simulink model "TOAD_Controller"  (R2025b)
settings: Solver=VariableStepAuto  StartTime=0.0  StopTime=10.0  RelTol=1e-3
undefined symbols (not defined in the file or in its folder): constantsASTRA, dt_SIM, u0
settings Model: Creator=pplat  LastModifiedBy=andrew

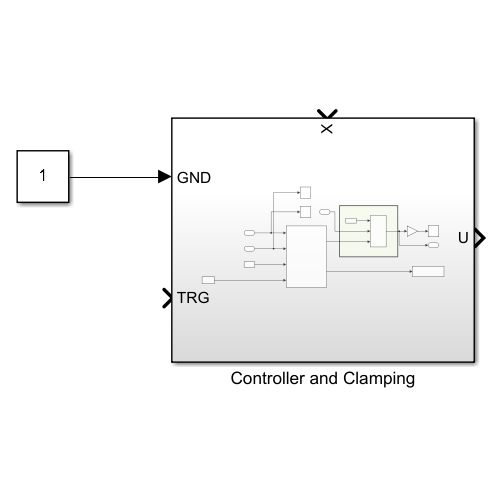
[thumbnail: Simulink's stored preview of the top-level diagram]
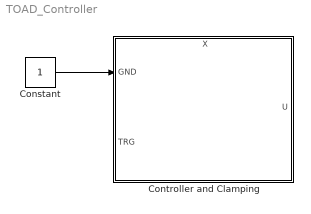
== system TOAD_Controller ==
  Constant : Constant
  Controller and Clamping : Subsystem
      settings: PortSchema="{\"entries\":[{\"content\":{\"sides\":[{\"content\":{\"connectorIds\":[\"In1\",\"In2\"]},\"type\":\"ConnectorPlacement.EquallySpacedRectSide\",\"uuid\":\"ecbe546b-cb94-472f-8bff-97599afc2d8a\"},{\"content\":{\"connectorIds\":[\"Out1\"],\"side\":\"RIGHT\"},\"type\":\"ConnectorPlacement.EquallySpacedRectSide\",\"uuid\":\"5863f614-a2a8-49af-9209-63f06ca85da1\"},{\"content\":{\"connectorIds\":[\"In3\"],\"side\":\"TOP\"},\"type\":\"ConnectorPlacement.EquallySpacedRectSide\",\"uuid\":\"6e100a99-a304-4bec-8fe0-0dacf7d0f0e2\"}]},\"type\":\"ConnectorPlacement.EquallySpacedConnector\",\"uuid\":\"0527d0f7-8d45-4b0a-99f9-95f3ca68c54e\"}],\"packageUris\":[\"http://schema.mathworks.com/mf0/Connector/R2020b\"],\"version\":\"1.0\"}"
  wires:
  Constant/1 -> Controller and Clamping/1(GND)

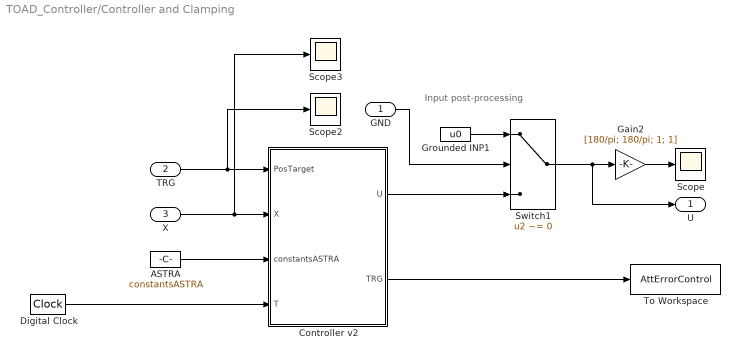
== system TOAD_Controller/Controller and Clamping ==
  note: Input post-processing
  GND : Inport
  TRG : Inport  Port=2
  X : Inport  Port=3
  ASTRA : Constant  Value=constantsASTRA  OutDataTypeStr=Bus: slBus1
  Controller v2 : MATLAB Function  TreatAsAtomicUnit=on
  Digital Clock : DigitalClock  SampleTime=dt_SIM
  Gain2 : Gain  Gain=[180/pi; 180/pi; 1; 1]
  Grounded INP1 : Constant  Value=u0
  Scope : Scope
      settings: ActiveDisplayYMinimum=-11.801195540279929  ActiveDisplayYMaximum=6.2107598625193638  DataLoggingVariableName=ScopeData9
  Scope2 : Scope
      settings: ActiveDisplayYMinimum=-1  ActiveDisplayYMaximum=1  DataLoggingVariableName=ScopeData18
  Scope3 : Scope
      settings: ActiveDisplayYMinimum=-0.53566092037557744  ActiveDisplayYMaximum=3.4212061004598149  DataLoggingVariableName=ScopeData19
  Switch1 : Switch  Criteria=u2 ~= 0  SaturateOnIntegerOverflow=off  InputSameDT=off
  To Workspace : ToWorkspace  VariableName=AttErrorControl  SaveFormat=Timeseries  SampleTime=-1
  U : Outport
  wires:
  Digital Clock/1 -> Controller v2/4(T)
  Controller v2/1(U) -> Switch1/3
  GND/1 -> Switch1/2
  Grounded INP1/1 -> Switch1/1
  Switch1/1 -> U/1, Gain2/1
  TRG/1 -> Scope2/1, Controller v2/1(PosTarget)
  X/1 -> Scope3/1, Controller v2/2(X)
  ASTRA/1 -> Controller v2/3(constantsASTRA)
  Gain2/1 -> Scope/1
  Controller v2/2(TRG) -> To Workspace/1

== matlab function TOAD_Controller/Controller and Clamping/Controller v2 ==
  data: PosTarget input; X input; constantsASTRA input; U output; T input; TRG output
function [U, TRG] = ControlFCN(PosTarget, X, constantsASTRA,  T)

    [U, TRG] = ASTRAv2_Controller(PosTarget, X, constantsASTRA,  T);
